simulink model "nonlinear_inverted_pendulum_simulation"  (R2016b)
settings: Solver=VariableStepAuto  StartTime=0.0  StopTime=10.0  RelTol=1e-3
values from neighbouring files (symbols this model uses):
  B = sys.B    [LoopGain.m]    (also in dcontrold_dir.m = sys_d.B; main.m = [                   0; ( 3*Km*Vs)/(LinkMass*(LinkLength^2)*R; simulation.m)
  Ctrl_FB = minreal( -tf( ss(A - L*C - B*K, L, K, zeros(nInputs,nOutputs))))    [simulation.m]
  g = 9.81    [main.m]
  Kb = Km    (= 0.0265805280355)    [main.m]
  Km = Vs/kappa_id    (= 0.0265805280355)    [main.m]    (also in sysStateEstimatorFeedbackWithModel.m = Kaug(nStates + 1:end))
  L = place(A',C',Lp)'    [dcontrold_dir.m]    (also in dcontrold_ind.m = place(A', C', desObsPoles).')
  Ts = sys.Ts    [LoopGain.m]    (also in analysis.m = 1/Hz; main.m = T(tdx); simulation.m = 0.001; system_id_batch.m = 0.001)
  Vs = 12    [main.m]
undefined symbols (not defined in the file or in its folder): Kc, m, Nc, R
libraries: cstblocks x3
settings Model: Creator=pong0923  LastModifiedBy=pong0923
settings DataIOCC: ExternalInput=[m]  LoadExternalInput=on

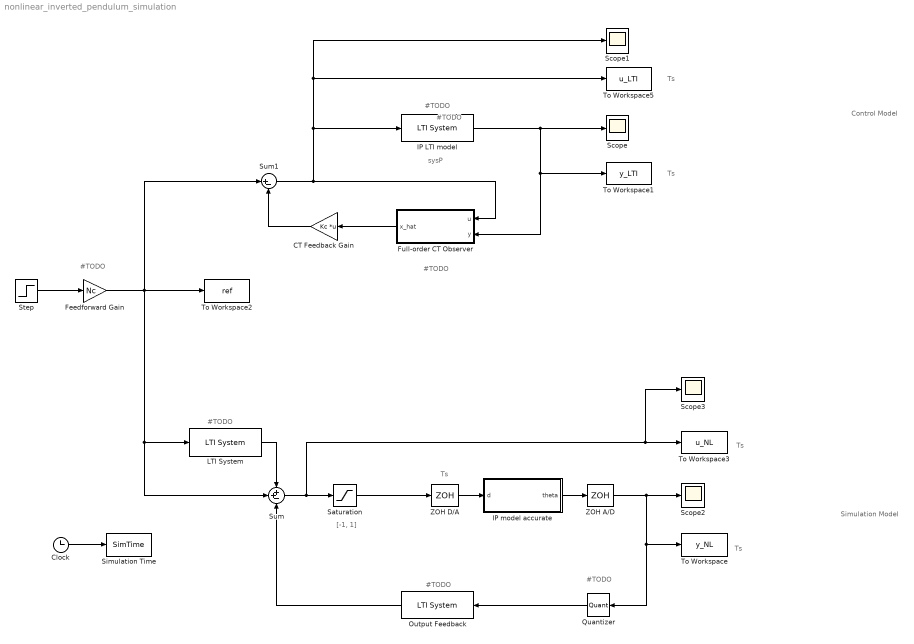
== system nonlinear_inverted_pendulum_simulation ==
  note: Simulation Model
  note: Control Model
  note: #TODO
  note: #TODO
  note: #TODO
  note: sysP
  note: Ts
  note: Ts
  note: #TODO
  note: #TODO
  note: [-1, 1]
  note: Ts
  note: #TODO
  note: #TODO
  note: Ts
  note: Ts
  CT Feedback Gain : Gain  Gain=Kc  Multiplication=Matrix(K*u)
  Clock : Clock
  Feedforward Gain : Gain  Gain=Nc
  Full-order CT Observer : Subsystem
  IP LTI model : cstblocks/LTI System  sys=sysP  IC=[]
  IP model accurate : Subsystem
  LTI System : cstblocks/LTI System  sys=Ctrl_FF  IC=[]
  Output Feedback : cstblocks/LTI System  sys=-Ctrl_FB  IC=[]
  Quantizer : Quantizer  QuantizationInterval=QzrLvl
  Saturation : Saturate  UpperLimit=1  LowerLimit=-1
  Scope{,1..3} (4 alike) : Scope
  Simulation Time : ToWorkspace  VariableName=SimTime  SampleTime=-1
  Step : Step  After=.1  SampleTime=0
  Sum : Sum  Inputs=++-
  Sum1 : Sum  Inputs=|+-
  To Workspace : ToWorkspace  VariableName=y_NL  SaveFormat=Timeseries  SampleTime=Ts
  To Workspace1 : ToWorkspace  VariableName=y_LTI  SaveFormat=Timeseries  SampleTime=Ts
  To Workspace2 : ToWorkspace  VariableName=ref  SaveFormat=Timeseries  SampleTime=-1
  To Workspace3 : ToWorkspace  VariableName=u_NL  SaveFormat=Timeseries  SampleTime=-1
  To Workspace5 : ToWorkspace  VariableName=u_LTI  SaveFormat=Timeseries  SampleTime=Ts
  ZOH A/D : ZeroOrderHold  SampleTime=Ts
  ZOH D/A : ZeroOrderHold  SampleTime=Ts
  wires:
  ZOH D/A/1 -> IP model accurate/1(d)
  IP model accurate/1(theta) -> ZOH A/D/1
  Clock/1 -> Simulation Time/1
  Saturation/1 -> ZOH D/A/1
  Sum/1 -> To Workspace3/1, Scope3/1, Saturation/1
  Step/1 -> Feedforward Gain/1
  Feedforward Gain/1 -> Sum1/1, LTI System/1, Sum/2, To Workspace2/1
  ZOH A/D/1 -> Quantizer/1, To Workspace/1, Scope2/1
  CT Feedback Gain/1 -> Sum1/2
  IP LTI model/1 -> Full-order CT Observer/2(y), To Workspace1/1, Scope/1
  Sum1/1 -> Full-order CT Observer/1(u), IP LTI model/1, To Workspace5/1, Scope1/1
  Full-order CT Observer/1(x_hat) -> CT Feedback Gain/1
  LTI System/1 -> Sum/1
  Quantizer/1 -> Output Feedback/1
  Output Feedback/1 -> Sum/3

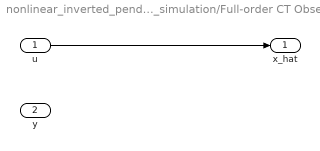
== system nonlinear_inverted_pendulum_simulation/Full-order CT Observer ==
  u : Inport
  y : Inport  Port=2
  x_hat : Outport
  wires:
  u/1 -> x_hat/1

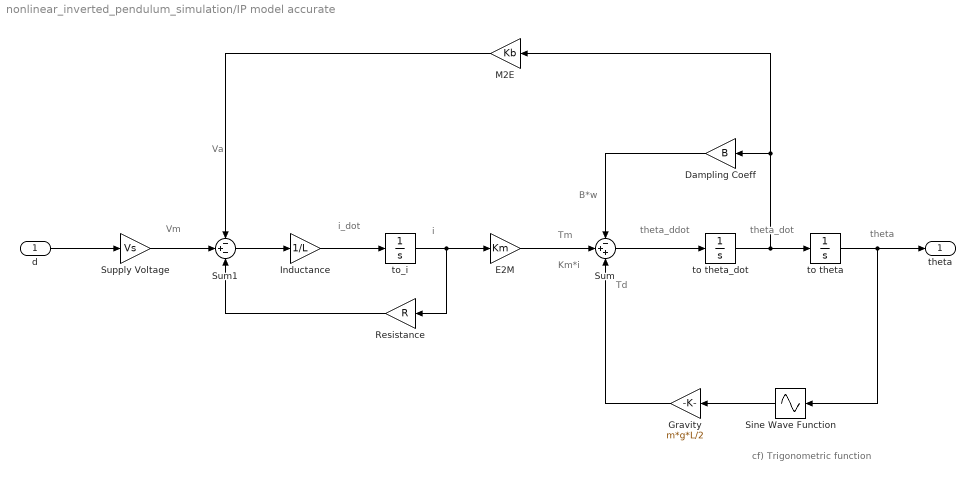
== system nonlinear_inverted_pendulum_simulation/IP model accurate ==
  note: Va
  note: Vm
  note: i_dot
  note: B*w
  note: Td
  note: Km*i
  note: Tm
  note: i
  note: cf) Trigonometric
      | function
  note: theta_ddot
  note: theta
  note: theta_dot
  d : Inport
  Dampling Coeff : Gain  Gain=B
  E2M : Gain  Gain=Km
  Gravity : Gain  Gain=m*g*L/2
  Inductance : Gain  Gain=1/L
  M2E : Gain  Gain=Kb
  Resistance : Gain  Gain=R
  Sine Wave Function : Sin  TimeSource=Use external signal  SampleTime=0
  Sum : Sum  Inputs=-++
  Sum1 : Sum  Inputs=-+-
  Supply Voltage : Gain  Gain=Vs
  to theta : Integrator
  to theta_dot : Integrator
  to_i : Integrator
  theta : Outport
  wires:
  to theta_dot/1 -> to theta/1, M2E/1, Dampling Coeff/1
  to theta/1 -> Sine Wave Function/1, theta/1
  Sine Wave Function/1 -> Gravity/1
  E2M/1 -> Sum/2
  Dampling Coeff/1 -> Sum/1
  Gravity/1 -> Sum/3
  to_i/1 -> Resistance/1, E2M/1
  Resistance/1 -> Sum1/3
  d/1 -> Supply Voltage/1
  Supply Voltage/1 -> Sum1/2
  M2E/1 -> Sum1/1
  Sum1/1 -> Inductance/1
  Inductance/1 -> to_i/1
  Sum/1 -> to theta_dot/1
